simulink model "TC_P1_C"  (R2014a)
settings: Solver=ode45  StartTime=0.0  StopTime=100  RelTol=1e-3
libraries: commrandsrc2 x1, commnoisgen2 x1, dsparch4 x1, commsink2 x1, dspsigops x1
settings Model: Creator=#sandaru  LastModifiedBy=root
settings DebuggingCC: MergeDetectMultiDrivingBlocksExec=error

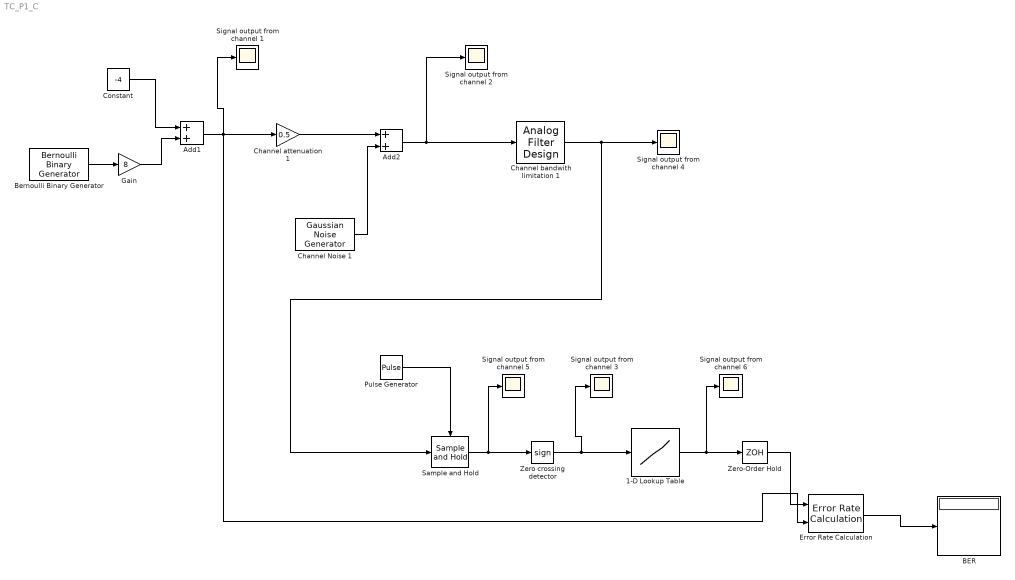
== system TC_P1_C ==
  1-D Lookup Table : Lookup_n-D  NumberOfTableDimensions=1  BreakpointsForDimension1=[-1 1]  Table=[-4 4]  InternalRulePriority=Speed  RndMeth=Simplest  InputSameDT=on
  Add1 : Sum
  Add2 : Sum
  "BER " : Display
  Bernoulli Binary Generator : commrandsrc2/Bernoulli Binary Generator  P=0.5  seed=61  Ts=0.1  frameBased=off  sampPerFrame=1  orient=off  outDataType=double
  Channel attenuation 1 : Gain  Gain=0.5
  Channel Noise 1 : commnoisgen2/Gaussian Noise Generator  m=0  d=2  s=41  Ts=0.01  frameBased=off  sampPerFrame=1  orient=off  outDataType=double
  Channel bandwith limitation 1 : dsparch4/Analog Filter Design  method=Butterworth  filttype=Lowpass  N=10  Wlo=1000  Whi=80  Rp=2  Rs=40
  Constant : Constant  Value=-4
  Error Rate Calculation : commsink2/Error Rate Calculation  N=1  st_delay=0  cp_mode=Entire frame  subframe=[]  PMode=Port  WsName=ErrorVec  RsMode2=off  stop=off  numErr=100  maxBits=1e6
  Gain : Gain  Gain=8
  Pulse Generator : DiscretePulseGenerator  PulseType=Time based  Period=0.1  PulseWidth=50
  Sample and Hold : dspsigops/Sample and Hold  trig=Rising edge  initCond=0  latchinput=off
  Signal output from channel {1..6} (6 alike) : Scope
      Signal output from channel 1 settings: SaveName=ScopeData5
      Signal output from channel 4 settings: SaveName=ScopeData2
      Signal output from channel 5 settings: SaveName=ScopeData3
      Signal output from channel 6 settings: SaveName=ScopeData4
  "Zero crossing detector " : Signum
  Zero-Order Hold : ZeroOrderHold  SampleTime=0.1
  wires:
  Bernoulli Binary Generator/1 -> Gain/1
  Gain/1 -> Add1/2
  Constant/1 -> Add1/1
  Add1/1 -> Error Rate Calculation/1, Signal output from channel 1/1, Channel attenuation 1/1
  Channel attenuation 1/1 -> Add2/1
  Channel Noise 1/1 -> Add2/2
  Add2/1 -> Signal output from channel 2/1, Channel bandwith limitation 1/1
  Channel bandwith limitation 1/1 -> Sample and Hold/1, Signal output from channel 4/1
  Pulse Generator/1 -> Sample and Hold/Trigger
  Sample and Hold/1 -> Signal output from channel 5/1, "Zero crossing detector "/1
  "Zero crossing detector "/1 -> Signal output from channel 3/1, 1-D Lookup Table/1
  1-D Lookup Table/1 -> Signal output from channel 6/1, Zero-Order Hold/1
  Zero-Order Hold/1 -> Error Rate Calculation/2
  Error Rate Calculation/1 -> "BER "/1
